simulink model "traffic_light_stream"  (R2022a)
settings: Solver=FixedStepDiscrete  StartTime=0.0  StopTime=inf  FixedStep=0.002  RelTol=1e-3  EnableMultiTasking=on
libraries: quarc_library x8
settings Model: ExtModeTrigDuration=10000  Creator=Lorena Gonzalez  LastModifiedBy=Lorena Gonzalez
settings SolverCC: AlgebraicLoopSolver=TrustRegion  PositivePriorityOrder=on
settings DataIOCC: ReturnWorkspaceOutputs=off
settings DebuggingCC: UnconnectedInputMsg=warning  UnconnectedOutputMsg=warning  UnconnectedLineMsg=warning  ArithmeticOperatorsInVariantConditions=warning
settings SFSimCC: SimUseLocalCustomCode=off  CustomCodeUndefinedFunction=UseInterfaceOnly
settings RTWCC: Description=QUARC Win64 Target Using Toolchain  SystemTargetFile=quarc_win64.tlc  TemplateMakefile=quarc_default_tmf  RTWUseLocalCustomCode=off  Toolchain=QUARC win64 | nmake (64-bit Windows)  BuildConfiguration=Faster Runs
settings CodeAppCC: StateflowObjectComments=on
settings STFCustomTargetCC: TargetLangStandard=C99 (ISO)  ConcurrentExecutionCompliant=on  UseToolchainInfoCompliant=on  SystemTargetFile=quarc_win64.tlc
settings GRTTargetCC: ParMdlRefBuildCompliant=off  CompOptLevelCompliant=off  CombineOutputUpdateFcns=off  MatFileLogging=off  CPPClassGenCompliant=off  GRTInterface=on  ExtMode=on  ExtModeMexFile=quarc_comm  ExtModeMexArgs='-w -d %d -uri %u -IP_TrafficLight 192.168.2.3','tcpip://localhost:17010'
settings ConfigComp: CovMetricSettings=dswe

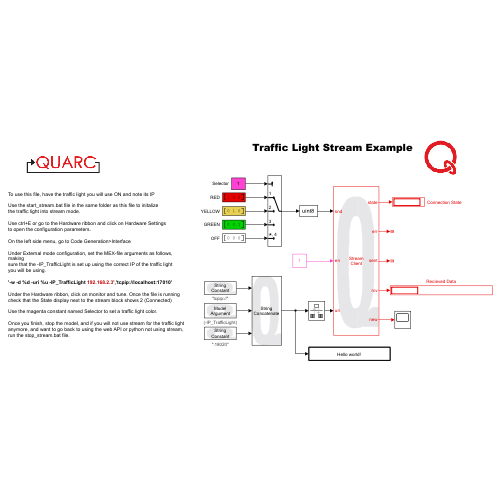
[thumbnail: Simulink's stored preview of the top-level diagram]
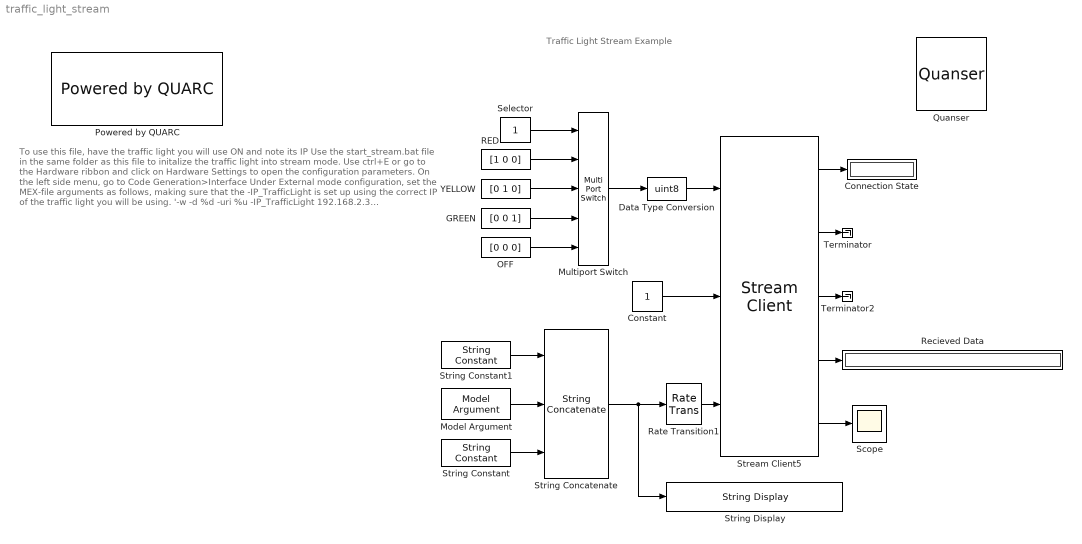
== system traffic_light_stream ==
  note: Traffic Light Stream Example
  note: To use this file, have the traffic light you will use ON and note its IP
      |
      | Use the start_stream.bat file in the same folder as this file to initalize
      | the traffic light into stream mode.
      |
      | Use ctrl+E or go to the Hardware ribbon and click on Hardware Settings
      | to open the configuration parameters.
      |
      | On the left side menu, go to Code Generation>Interface
      |
      | Under External mode configuration, set the MEX-file arguments as follows, making
      | sure that the -IP_TrafficLight is set up using the correct IP of the traffic light
      | you will be using.
      |
      | '-w -d %d -uri %u -IP_TrafficLight 192.168.2.3 ','tcpip://localhost:17010'
      |
      | Under the Hardware ribbon, click on monitor and tune. Once the file is running
      | check that the State display next to the stream block shows 2 (Connected)
      |
      | Use the magenta constant named Selector to set a traffic light color.
      |
      | Once you finish, stop the model, and if you will not use stream for the traffic light anymore, and want to go back to using the web API or python not using stream,
      | run the stop_stream.bat file.
  Connection State : Display
  Constant : Constant
  Data Type Conversion : DataTypeConversion  OutDataTypeStr=uint8  SaturateOnIntegerOverflow=off  RndMeth=Floor
  GREEN : Constant  Value=[0 0 1]
  Model Argument : quarc_library/Sources/Signals/Model Argument  argument_name=IP_TrafficLight  has_value=on  data_type_mode=Specify via dialog  data_type=char  max_length=80  default_value=0  default_string=192.168.2.3  variable_size=off
      settings: AttributesFormatString=(-%<argument_name>)  SourceProductName=QUARC Targets
  Multiport Switch : MultiPortSwitch  Inputs=4  DiagnosticForDefault=None  SaturateOnIntegerOverflow=off  InputSameDT=off
  OFF : Constant  Value=[0 0 0]
  Powered by QUARC : quarc_library/Logos/Powered by QUARC
  Quanser : quarc_library/Logos/Quanser
  RED : Constant  Value=[1 0 0]
  Rate Transition1 : RateTransition
  Recieved Data : Display
  Scope : Scope
  Selector : Constant
  Stream Client5 : quarc_library/Communications/Basic/Stream Client  uri_source=External input port  uri=tcpip://192.168.1.20:18020  send_buffer_size=1460  receive_buffer_size=1460  byte_order=little endian (Intel - LSB first)  optimization=Minimum latency  send_options=Send most recent data  receive_options=Receive most recent data  default_value=uint8([0 0 0])  sample_time=.1  active=off  implementation=Use blocking I/O in a separate thread  send_fifo_size=1000  receive_fifo_size=1000  send_priority=0  receive_priority=0  send_dimensions=off  receive_dimensions=off  max_dimensions=-1  data_type=uint8  type_expr=BusObject
  String Concatenate : quarc_library/Strings/String Concatenate  num_inputs=3  max_length=0  output_size=Inherit from input
      settings: SourceProductName=QUARC Targets
  String Constant : quarc_library/Strings/String Constant  string_value=:18020  evaluate_string=off  string_type=text  max_length=80  sample_time=inf  variable_size=off
      settings: AttributesFormatString="\":18020\""  SourceProductName=QUARC Targets
  String Constant1 : quarc_library/Strings/String Constant  string_value=tcpip://  evaluate_string=off  string_type=text  max_length=80  sample_time=inf  variable_size=off
      settings: AttributesFormatString="\"tcpip://\""  SourceProductName=QUARC Targets
  String Display : quarc_library/Strings/String Display  alignment=center  display_mode=Single line  sample_time=-1  use_new=off
      settings: SourceProductName=QUARC Targets
  Terminator : Terminator
  Terminator2 : Terminator
  YELLOW : Constant  Value=[0 1 0]
  wires:
  Stream Client5/1 -> Connection State/1
  Stream Client5/3 -> Terminator2/1
  Constant/1 -> Stream Client5/2
  Stream Client5/2 -> Terminator/1
  Model Argument/1 -> String Concatenate/2
  String Constant/1 -> String Concatenate/3
  String Constant1/1 -> String Concatenate/1
  Stream Client5/4 -> Recieved Data/1
  Stream Client5/5 -> Scope/1
  String Concatenate/1 -> String Display/1, Rate Transition1/1
  Rate Transition1/1 -> Stream Client5/3
  Multiport Switch/1 -> Data Type Conversion/1
  OFF/1 -> Multiport Switch/5
  GREEN/1 -> Multiport Switch/4
  YELLOW/1 -> Multiport Switch/3
  RED/1 -> Multiport Switch/2
  Selector/1 -> Multiport Switch/1
  Data Type Conversion/1 -> Stream Client5/1
